simulink model "threedof"  (R2022b)
settings: Solver=VariableStepAuto  StartTime=0.0  StopTime=10  RelTol=1e-3
values from neighbouring files (symbols this model uses):
  Gimbal_offset_X = randn*0.0174533*0.33    [montecarlo3dof.m]
undefined symbols (not defined in the file or in its folder): DiscIntNeverNeededParam, magnitude, sigbuilder_block
libraries: simulink x1
settings Model: Creator=Freddie  LastModifiedBy=Freddie

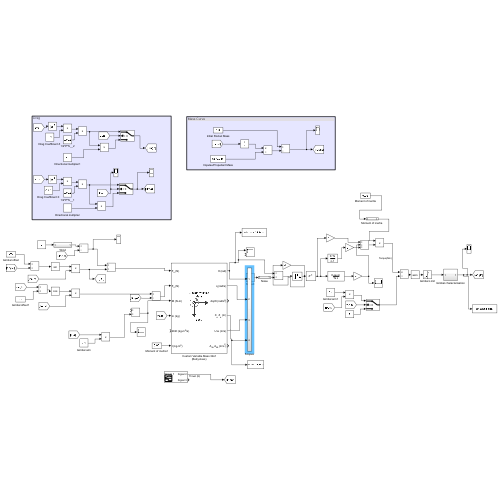
[thumbnail: Simulink's stored preview of the top-level diagram]
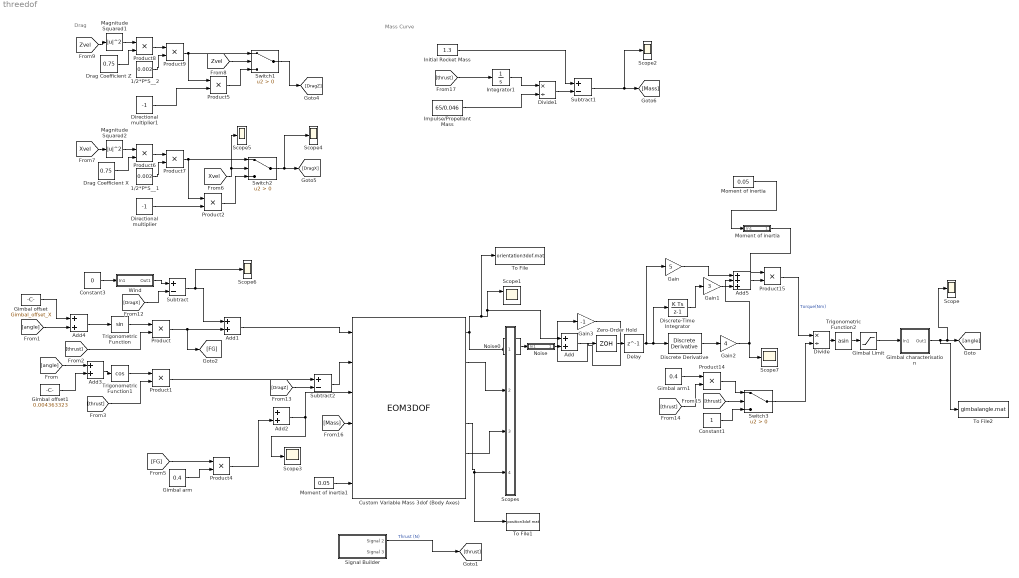
== system threedof ==
  note: Mass Curve
  note: Drag
  1/2*P*S__1 : Constant  Value=0.002
  1/2*P*S__2 : Constant  Value=0.002
  Add{,1..4} (5 alike) : Sum
  Add5 : Sum  Inputs=+++
  Constant1 : Constant
  Constant3 : Constant  Value=0
  Custom Variable Mass 3dof (Body Axes) : EOM3DOF  mtype=Custom Variable  v_ini=0  mass=1.3  mass_e=1.254  mass_f=1.3  Iyy=0.05  Iyy_e=0.0000001  Iyy_f=0.05  g=-9.81
  Delay : Delay  DelayLength=1  InitialCondition=0
  Directional multiplier : Constant  Value=-1
  Directional multiplier1 : Constant  Value=-1
  Discrete Derivative : simulink/Quick Insert/Discrete/Discrete Derivative  gainval=1  ICPrevScaledInput=0.0  OutMin=[]  OutMax=[]  OutDataType=fixdt(1, 16)  OutScaling=2^-10  DoSatur=off
  Discrete-Time Integrator : DiscreteIntegrator  SampleTime=0.1  ICPrevOutput=DiscIntNeverNeededParam  ICPrevScaledInput=DiscIntNeverNeededParam
  Divide : Product  Inputs=*/
  Divide1 : Product  Inputs=*/
  Drag Coefficient X : Constant  Value=0.75
  "Drag Coefficient Z " : Constant  Value=0.75
  Gain : Gain  Gain=5
  Gain1 : Gain  Gain=3
  Gain2 : Gain  Gain=4
  Gain3 : Gain  Gain=-1
  Gimbal Limit : Saturate  UpperLimit=0.139626  LowerLimit=-0.139626
  Gimbal arm : Constant  Value=0.4
  Gimbal arm1 : Constant  Value=0.4
  Gimbal characterisation : Subsystem
  Gimbal offset : Constant  Value=Gimbal_offset_X
  Gimbal offset1 : Constant  Value=0.004363323
  Impulse/Propellant Mass : Constant  Value=65/0.046
  Initial Rocket Mass : Constant  Value=1.3
  Integrator1 : Integrator
  Magnitude Squared1 : Math  Operator=magnitude^2
  Magnitude Squared2 : Math  Operator=magnitude^2
  Moment of inertia : Constant  Value=0.05
  "Moment of inertia " : Subsystem
  Moment of inertia1 : Constant  Value=0.05
  Noise : Subsystem
  Noise0 : Constant  Value=0
  Product{,1..2,4..9,14..15} (11 alike) : Product
  Scope{,2..7} (7 alike) : Scope
  Scope1 : Scope  NumInputPorts=2
  Scopes : Subsystem
  Signal Builder : Subsystem  Tag=STV Subsys  LoadFcn=sigbuilder_block('load');  StartFcn=sigbuilder_block('start');  StopFcn=sigbuilder_block('stop');  ClipboardFcn=sigbuilder_block('clipboard');  mask(Sigbuilder block){tuvar=[0:10]}
      mask help: Simulink:masks:SigbuilderBlock_MD
      mask init:
      | if ~strcmp(get_param(bdroot(gcbh),'SimulationStatus'),'stopped') tuvar = sigbuilder_block('maskInit'); end
      settings: CopyFcn=sigbuilder_block('copy');  DeleteFcn=sigbuilder_block('delete');  ModelCloseFcn=sigbuilder_block('modelClose');  PreSaveFcn=sigbuilder_block('preSave');  PauseFcn=sigbuilder_block('pause');  ContinueFcn=sigbuilder_block('continue');  NameChangeFcn=sigbuilder_block('namechange');  OpenFcn=sigbuilder_block('open',[437.6 199.2 550.4 400 ]);  CloseFcn=sigbuilder_block('close');
      mask Display: plot(0, 0, 100, 100,[2, 2, 32, 32, 2], [68, 8, 8, 68, 68],[32, 2], [38, 38], [32, 19, 2],[53, 60, 44], [32, 17, 17, 2],[16, 16, 31, 31]);txt = getActiveGroup(gcbh);text(2, 100, txt,'verticalAlignment', 'top');
  Subtract : Sum  Inputs=+-
  Subtract1 : Sum  Inputs=+-
  Subtract2 : Sum  Inputs=+-
  Switch1 : Switch  Criteria=u2 > Threshold  SaturateOnIntegerOverflow=off  InputSameDT=off
  Switch2 : Switch  Criteria=u2 > Threshold  SaturateOnIntegerOverflow=off  InputSameDT=off
  Switch3 : Switch  Criteria=u2 > Threshold  SaturateOnIntegerOverflow=off  InputSameDT=off
  To File : ToFile  Filename=orientation3dof.mat  MatrixName=orientation  SampleTime=0.05
  To File1 : ToFile  Filename=position3dof.mat  MatrixName=position  SampleTime=0.05
  To File2 : ToFile  Filename=gimbalangle.mat  MatrixName=angle  SampleTime=0.01
  Trigonometric Function : Trigonometry
  Trigonometric Function1 : Trigonometry  Operator=cos
  Trigonometric Function2 : Trigonometry  Operator=asin
  Wind : Subsystem
  Zero-Order Hold : ZeroOrderHold  SampleTime=0.01
  wires:
  Signal Builder/1(Signal 2) -> [thrust]  "Thrust (N)"
  Trigonometric Function/1 -> Product/1
  [thrust] -> Product/2
  Trigonometric Function1/1 -> Product1/1
  Product/1 -> [FG], Add1/2
  [FG] -> Product4/1
  Gimbal arm/1 -> Product4/2
  Add2/1 -> Custom Variable Mass 3dof (Body Axes)/3, Scope3/1
  Product4/1 -> Add2/2
  Custom Variable Mass 3dof (Body Axes)/1 -> Scopes/1(In2), To File/1, Scope1/1, Add/1
  Custom Variable Mass 3dof (Body Axes)/2 -> Scopes/2(In3)
  Custom Variable Mass 3dof (Body Axes)/4 -> To File1/1, Scopes/4(In1)
  Noise/1(Out1) -> Add/2
  Gimbal characterisation/1(Out1) -> To File2/1, Scope/1, [angle]
  Noise0/1 -> Noise/1(In1)
  Custom Variable Mass 3dof (Body Axes)/5 -> Scopes/3(In4)
  Constant3/1 -> Wind/1(In1)
  [Xvel] -> Scope5/1, Switch2/2
  [Xvel] -> Magnitude Squared2/1
  Product7/1 -> Product2/1, Switch2/1
  Magnitude Squared2/1 -> Product6/1
  Drag Coefficient X/1 -> Product6/2
  Product6/1 -> Product7/1
  1/2*P*S__1/1 -> Product7/2
  Subtract2/1 -> Custom Variable Mass 3dof (Body Axes)/2
  Switch2/1 -> Scope4/1, [DragX]
  Product1/1 -> Subtract2/1
  [DragZ] -> Subtract2/2
  Wind/1(Out1) -> Subtract/1
  [DragX] -> Subtract/2
  Subtract/1 -> Scope6/1, Add1/1
  Add1/1 -> Custom Variable Mass 3dof (Body Axes)/1
  Gimbal arm1/1 -> Product14/1
  [thrust] -> Product14/2
  Divide/1 -> Trigonometric Function2/1
  Trigonometric Function2/1 -> Gimbal Limit/1
  Switch3/1 -> Divide/2
  Product14/1 -> Switch3/1
  [thrust] -> Switch3/2
  Constant1/1 -> Switch3/3
  Product15/1 -> Divide/1  "Torque(Nm)"
  Moment of inertia/1 -> "Moment of inertia "/1(In1)
  Add4/1 -> Trigonometric Function/1
  [angle] -> Add4/2
  Gimbal offset/1 -> Add4/1
  "Moment of inertia "/1(Out1) -> Product15/1
  [Mass] -> Custom Variable Mass 3dof (Body Axes)/4
  [angle] -> Add3/1
  Add3/1 -> Trigonometric Function1/1
  Gimbal offset1/1 -> Add3/2
  [thrust] -> Product1/2
  Gimbal Limit/1 -> Gimbal characterisation/1(In1)
  Directional multiplier/1 -> Product2/2
  Product2/1 -> Switch2/3
  Directional multiplier1/1 -> Product5/2
  Product5/1 -> Switch1/3
  Magnitude Squared1/1 -> Product8/1
  Product9/1 -> Product5/1, Switch1/1
  [Zvel] -> Magnitude Squared1/1
  1/2*P*S__2/1 -> Product9/2
  Switch1/1 -> [DragZ]
  Product8/1 -> Product9/1
  "Drag Coefficient Z "/1 -> Product8/2
  [Zvel] -> Switch1/2
  Initial Rocket Mass/1 -> Subtract1/1
  Impulse/Propellant Mass/1 -> Divide1/2
  Subtract1/1 -> Scope2/1, [Mass]
  [thrust] -> Integrator1/1
  Divide1/1 -> Subtract1/2
  Integrator1/1 -> Divide1/1
  Moment of inertia1/1 -> Custom Variable Mass 3dof (Body Axes)/6
  Zero-Order Hold/1 -> Delay/1
  Delay/1 -> Gain/1, Discrete-Time Integrator/1, Discrete Derivative/1
  Add5/1 -> Product15/2
  Gain/1 -> Add5/1
  Discrete-Time Integrator/1 -> Gain1/1
  Gain1/1 -> Add5/2
  Discrete Derivative/1 -> Gain2/1
  Gain2/1 -> Scope7/1, Add5/3
  Add/1 -> Gain3/1
  Gain3/1 -> Zero-Order Hold/1

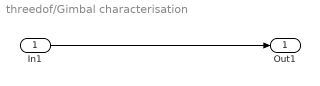
== system threedof/Gimbal characterisation ==
  In1 : Inport
  Out1 : Outport
  wires:
  In1/1 -> Out1/1

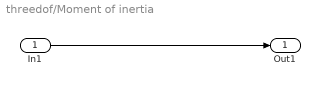
== system threedof/Moment of inertia  ==
  In1 : Inport
  Out1 : Outport
  wires:
  In1/1 -> Out1/1

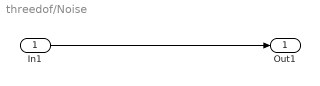
== system threedof/Noise ==
  In1 : Inport
  Out1 : Outport
  wires:
  In1/1 -> Out1/1

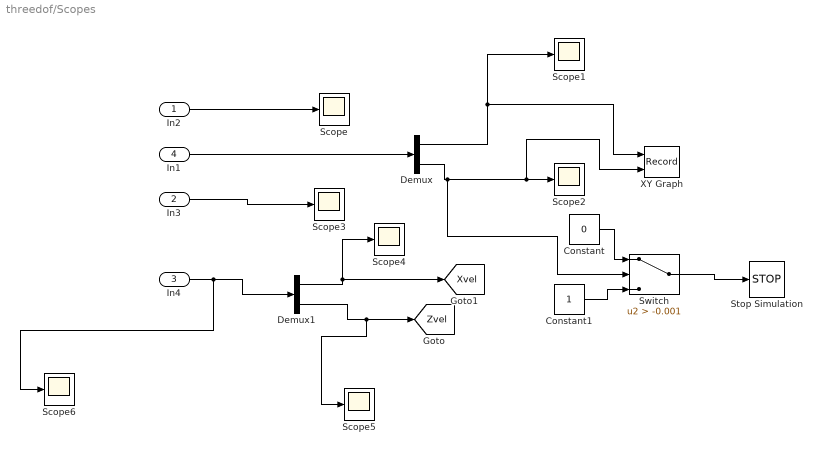
== system threedof/Scopes ==
  In2 : Inport
  In3 : Inport  Port=2
  In4 : Inport  Port=3
  In1 : Inport  Port=4
  Constant : Constant  Value=0
  Constant1 : Constant
  Demux : Demux  Outputs=2
  Demux1 : Demux  Outputs=2
  Scope{,1..6} (7 alike) : Scope
  Stop Simulation : Stop
  Switch : Switch  Criteria=u2 > Threshold  Threshold=-0.001  SaturateOnIntegerOverflow=off  InputSameDT=off
  XY Graph : Record  FileSettingsInternal="{\"entries\":[{\"content\":{\"excelSettings\":{\"content\":{},\"type\":\"Streamout.ExcelSettings\"}},\"type\":\"Streamout.FileSettingStorage\",\"uuid\":\"a2261c10-562a-4bfc-a90e-63c4fbe8525c\"}],\"packageUris\":[\"http://schema.mathworks.com/mf0/streamout_blocks/R2020a\"],\"version\":\"1.0\"}"  Layout=[1 1]  SignalsInternal="{\"entries\":[{\"content\":{\"signals\":[{\"content\":{\"blockPath\":[\"threedof/Scopes/XY Graph\"],\"channel\":[],\"dimensions\":[1],\"domain\":\"threedof/Scopes/XY Graph\",\"lineColor\":\"#a2142f\",\"plots\":[1],\"port\":1,\"sid\":[\"\"],\"signalID\":4614,\"signalName\":\"Demux:1\"},\"type\":\"RecordBlkView.Signal\",\"uuid\":\"29096a7a-50a4-45cf-941e-207e67bbf3e9\"},{\"content\":{\"blockPath\":[\"threedof/Scopes/XY Graph\"],\"channel\":[],\"dimensions\":[1],\"domain\":\"threedof/Scopes/XY Graph\",\"lineColor\":\"#139fff\",\"plots\":[1],\"port\":2,\"sid\":[\"\"],\"signalID\":4618,\"signalName\":\"Demux:2\"},\"type\":\"RecordBlkView.Signal\",\"uuid\":\"15fef38c-1e07-4efd-9cb6-25df3cede9e7\"}]},\"type\":\"RecordBlkView.InputSignals\",\"uuid\":\"30fdf703-fa63-46b5-9dae-05d990e43b76\"}],\"packageUris\":[\"http://schema.mathworks.com/mf0/streamout_blocks/R2020a\"],\"version\":\"1.0\"}"  VisualizationBindings="{\"xyplotplugin\":{\"info\":[{\"series\":[{\"bindingParametersList\":[{\"parameter\":\"X-Axis\",\"signalID\":4614,\"signalName\":\"Demux:1\"},{\"parameter\":\"Y-Axis\",\"signalID\":4618,\"signalName\":\"Demux:2\"}],\"seriesID\":26488}],\"subplotID\":1}]}}"  CompatibilityTag=XY
  tag scope: Xvel=global, Zvel=global
  wires:
  In2/1 -> Scope/1
  In1/1 -> Demux/1
  Demux/1 -> XY Graph/1, Scope1/1
  In3/1 -> Scope3/1
  In4/1 -> Scope6/1, Demux1/1
  Demux1/2 -> Scope5/1, [Zvel]
  Demux1/1 -> [Xvel], Scope4/1
  Demux/2 -> XY Graph/2, Scope2/1, Switch/2
  Switch/1 -> Stop Simulation/1
  Constant/1 -> Switch/1
  Constant1/1 -> Switch/3

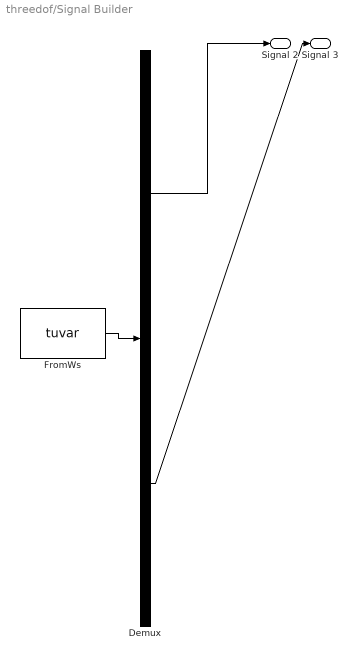
== system threedof/Signal Builder ==
  Demux : Demux  Tag=STV Demux  Outputs=2
      settings: DisplayOption=none
  FromWs : FromWorkspace  Tag=STV FromWs  VariableName=tuvar
      SigBuilderData=|
      | common.afterFinalStr = 'Extrapolate'
      | common.sampleTime = 0
      | dataSet.timeRange = [0 10]
      | dataSet.name = 'Group 1'
      | sbobj.Groups.Name = 'Group 1'
      | sbobj.Groups.Signals(1).Name = 'Signal 2'
      | sbobj.Groups.Signals(1).XData = [0 0.014 0.075 0.157 0.293 0.382 0.45 0.539 0.614 0.662 0.771 0.948 0.996 1.078 1.187 1.289 1.337 1.412 1.474 1.515 1.542 1.706 1.938 2.101 2.129 2.251 2.402 2.64 2.961 3.31 10]
      | sbobj.Groups.Signals(1).YData = [11.527 11.527 20.126 26.572 29.113 30.278 29.69 30.667 30.089 31.15 30.478 29.89 28.714 28.136 27.738 26.761 26.96 25.984 25.008 26.173 24.808 22.856 20.903 18.173 19.338 16.21 13.48 8.791 3.32 0 0]
      | sbobj.Groups.Signals(2).Name = 'Signal 3'
      | sbobj.Groups.Signals(2).XData = [0 3.31 10]
      | sbobj.Groups.Signals(2).YData = [1.3 1.254 1.254]
  Signal 2 : Outport  Tag=STV Outport
  Signal 3 : Outport  Tag=STV Outport  Port=2
  wires:
  FromWs/1 -> Demux/1
  Demux/1 -> Signal 2/1
  Demux/2 -> Signal 3/1

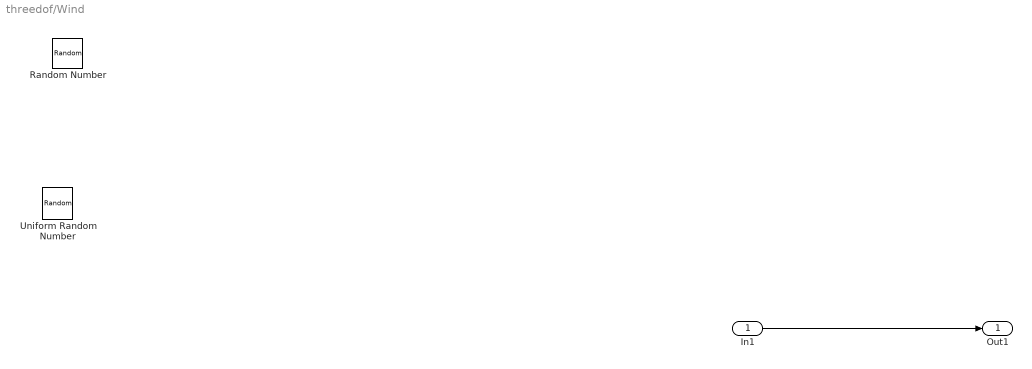
== system threedof/Wind ==
  In1 : Inport
  Random Number : RandomNumber  SampleTime=0.1
  Uniform Random Number : UniformRandomNumber  SampleTime=0.1
  Out1 : Outport
  wires:
  In1/1 -> Out1/1
